simulink model "ActuatorTest_ExampleI"  (Simulink 2.20)
settings: Solver=ode4  StartTime=0.0  StopTime=50  FixedStep=0.0025  RelTol=1e-3  AbsTol=1e-6
libraries: DABLib x3
settings Model: ConsistencyChecking=off  RTWPlaceOutputsASAP=off

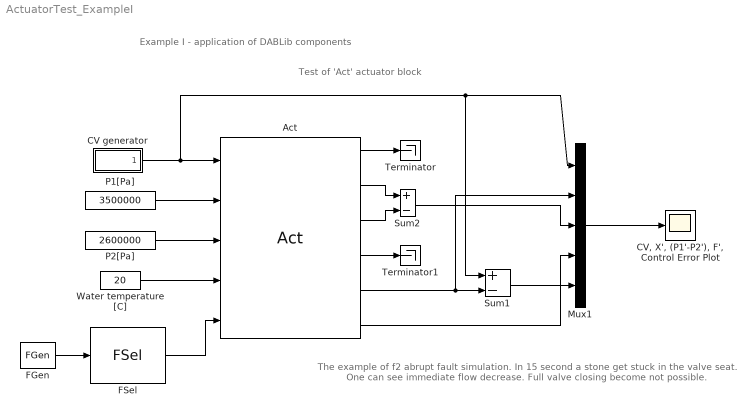
== system ActuatorTest_ExampleI ==
  note: Test of 'Act' actuator block
  note: Example I - application of DABLib components
  note: The example of f2 abrupt fault simulation.
      | In 15 second a stone get stuck in the valve seat.
      | One can see immediate flow decrease.
      |  Full valve closing become not possible.
  Act : DABLib/Act  Dist=off
  CV generator : Subsystem
  "CV, X', (P1'-P2'), F', Control Error Plot" : Scope
      settings: TickLabels=on  TimeRange=auto  YMin=0  YMax=1  SaveToWorkspace=off  SaveName=ScopeData  LimitMaxRows=off
  FGen : DABLib/FGen  From=15  To=inf  MFS=1  FDT=0  FSD=1
  FSel : DABLib/FSel  FSel=f2 - Valve plug or valve seat sedimentation
  Mux1 : Mux  Inputs=5
  "P1[Pa] " : Constant  Value=3500000
  "P2[Pa] " : Constant  Value=2600000
  Sum1 : Sum  Inputs=+-
  Sum2 : Sum  Inputs=+-
  Terminator : Terminator
  Terminator1 : Terminator
  Water temperature [C] : Constant  Value=20
  wires:
  Mux1/1 -> "CV, X', (P1'-P2'), F', Control Error Plot"/1
  FGen/1 -> FSel/1
  Sum2/1 -> Mux1/3
  CV generator/1(CV[0-1]) -> Sum1/1, Mux1/1, Act/1
  "P1[Pa] "/1 -> Act/2
  "P2[Pa] "/1 -> Act/3
  Water temperature [C]/1 -> Act/4
  Act/2 -> Sum2/1
  Act/3 -> Sum2/2
  Act/4 -> Terminator1/1
  Act/6 -> Mux1/4
  Act/5 -> Sum1/2, Mux1/2
  Act/1 -> Terminator/1
  Sum1/1 -> Mux1/5
  FSel/1 -> Act/5

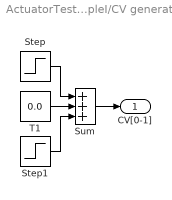
== system ActuatorTest_ExampleI/CV generator ==
  Step : Step  Time=0  Before=0  After=0.5
  Step1 : Step  Time=25  Before=0  After=0.5
  Sum : Sum  Inputs=+++
  T1 : Constant  Value=0.0
  CV[0-1] : Outport  Port=1  InitialOutput=0
  wires:
  Step/1 -> Sum/1
  T1/1 -> Sum/2
  Step1/1 -> Sum/3
  Sum/1 -> CV[0-1]/1
